simulink model "DCM_17_Series_18Ms_For_R_Discharge"  (R2019b)
settings: Solver=VariableStepAuto  StartTime=0.0  StopTime=30  RelTol=1e-3
model workspace (MAT data in the model file):
  Laf = 0.015
  Laf_2 = 0.00844
  Rarm = 0.0096
  angular_vel = 165
  angular_vel_1 = 175.405
  angular_vel_10 = 168.703
  angular_vel_11 = 168.598
  angular_vel_12 = 167.865
  angular_vel_13 = 167.132
  angular_vel_14 = 166.923
  angular_vel_15 = 165.666
  angular_vel_16 = 164.41
  angular_vel_2 = 173.625
  angular_vel_3 = 172.787
  angular_vel_4 = 170.902
  angular_vel_5 = 170.902
  angular_vel_6 = 169.96
  angular_vel_7 = 169.855
  angular_vel_8 = 169.122
libraries: powerlib x20, simulink x1
settings Model: OrderedModelArguments=off  Creator=Sy2  LastModifiedBy=Sy2
settings SolverCC: ZeroCrossAlgorithm=Adaptive
settings DebuggingCC: IgnoredZcDiagnostic=none

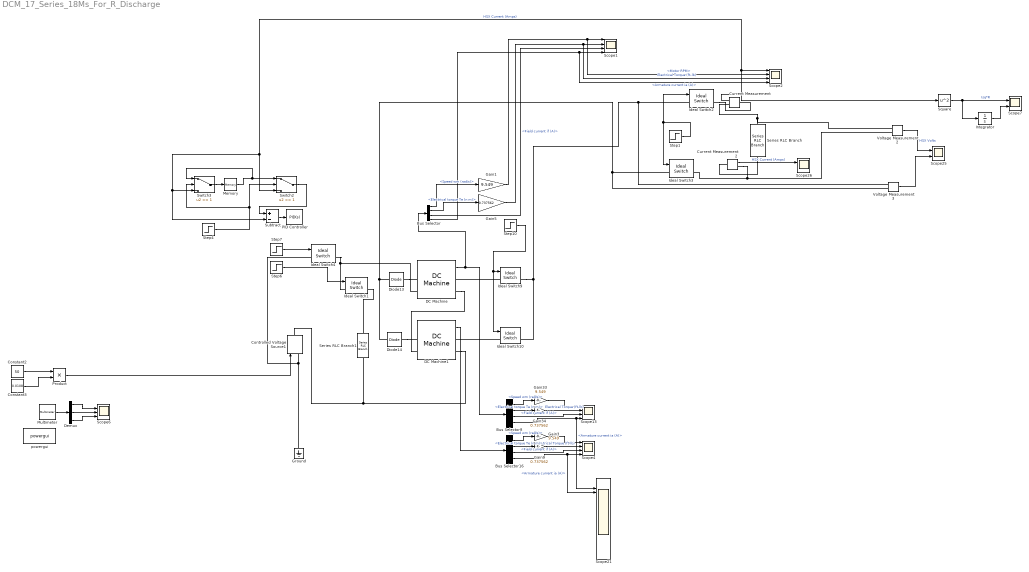
== system DCM_17_Series_18Ms_For_R_Discharge ==
  Bus Selector : BusSelector  OutputSignals=Speed wm (rad/s),Electrical torque Te (n m),Field current if (A),Armature current ia (A)
  Bus Selector16 : BusSelector  OutputSignals=Speed wm (rad/s),Electrical torque Te (n m),Field current if (A),Armature current ia (A)
  Bus Selector8 : BusSelector  OutputSignals=Speed wm (rad/s),Electrical torque Te (n m),Field current if (A),Armature current ia (A)
  Constant2 : Constant  Value=50
  Constant3 : Constant  Value=0.0108
  Controlled Voltage Source1 : powerlib/Electrical Sources/Controlled Voltage Source  Initialize=on  Source_Type=DC  Amplitude=0  Phase=0  Frequency=0  Measurements=Voltage
      settings: SourceProductName=Simscape Electrical
  Current Measurement : powerlib/Measurements/Current Measurement  PhasorSimulation=off  OutputType=Complex  PSBequivalent=0
      settings: SourceProductName=Simscape Electrical
  Current Measurement2 : powerlib/Measurements/Current Measurement  PhasorSimulation=off  OutputType=Complex  PSBequivalent=0
      settings: SourceProductName=Simscape Electrical
  DC Machine : powerlib/Machines/DC Machine  PresetModel=No  MechanicalLoad=Torque TL  FieldType=Wound  ShowDetailedParameters=on  MeasurementBus=off  RLa="[Rarm  0.002]"  RLf=[0.0054 0.0125]  Laf=Laf  MachineConstant=Torque constant (N.m/A)  Ke=1.8  Kt=1.8  J=137  Bm=0  Tf=0  w0=angular_vel  Ifinit=0  TsPowergui=0  TsBlock=-1
      settings: SourceProductName=Simscape Electrical
  DC Machine1 : powerlib/Machines/DC Machine  PresetModel=No  MechanicalLoad=Torque TL  FieldType=Wound  ShowDetailedParameters=on  MeasurementBus=off  RLa="[Rarm  0.002]"  RLf=[0.0054 0.0125]  Laf=Laf  MachineConstant=Torque constant (N.m/A)  Ke=1.8  Kt=1.8  J=137  Bm=0  Tf=0  w0=angular_vel  Ifinit=0  TsPowergui=0  TsBlock=-1
      settings: SourceProductName=Simscape Electrical
  Demux : Demux  Outputs=3
  Diode13 : powerlib/Power Electronics/Diode  Ron=0.0000001  Lon=0  Vf=0.8  IC=0  UseSnubber=0  Rs=500000  Cs=250e-9  Measurements=off
      settings: SourceProductName=Simscape Electrical
  Diode14 : powerlib/Power Electronics/Diode  Ron=0.001  Lon=0  Vf=0.8  IC=0  UseSnubber=0  Rs=500000  Cs=250e-9  Measurements=off
      settings: SourceProductName=Simscape Electrical
  Gain1 : Gain  Gain=9.549
  Gain3 : Gain  Gain=9.549
  Gain33 : Gain  Gain=9.549
  Gain34 : Gain  Gain=0.737562
  Gain5 : Gain  Gain=0.737562
  Gain9 : Gain  Gain=0.737562
  Ground : powerlib/Elements/Ground  LConnTagsString=a
      settings: SourceProductName=Simscape Electrical
  Ideal Switch{1..3,9..10} (5 alike) : powerlib/Power Electronics/Ideal Switch  Ron=0  Lon=0  IC=0  Rs=inf  Cs=0  Measurements=on
      settings: SourceProductName=Simscape Electrical
  Ideal Switch4 : powerlib/Power Electronics/Ideal Switch  Ron=0  Lon=0  IC=1  Rs=inf  Cs=0  Measurements=on
      settings: SourceProductName=Simscape Electrical
  Integrator : Integrator  ZeroCross=off
  Memory : Memory
  Multimeter : powerlib/Measurements/Multimeter  PhasorSimulation=off  OutputType=Complex  sel=[2 3 1]  L=3  Gain=[1 1 1]  yselected={'Usrc: Controlled Voltage Source1','Ib: Series RLC Branch1','Ub: Series RLC Branch1'};  PSBOutputType=1  PSBequivalent=0  AxesSetting=[0,0.1,-100,100]  Display=0  SavedBlockNames=-11
      settings: SourceProductName=Simscape Electrical
  PID Controller : simulink/Continuous/PID Controller  Controller=PID  Form=Parallel  TimeDomain=Continuous-time  SampleTime=-1  IntegratorMethod=Forward Euler  FilterMethod=Forward Euler  ControllerParametersSource=internal  P=10  I=7  D=1  UseFilter=on  N=100  TunerSelectOption=Transfer Function Based (PID Tuner App)  InitialConditionSource=internal  InitialConditionForIntegrator=0  InitialConditionForFilter=0  DifferentiatorICPrevScaledInput=0  ExternalReset=none  TrackingMode=off  Kt=1  LimitOutput=off  UpperSaturationLimit=inf  LowerSaturationLimit=-inf  LinearizeAsGain=on  AntiWindupMode=none  Kb=1  POutMin=[]  POutMax=[]  IOutMin=[]  IOutMax=[]  DOutMin=[]  DOutMax=[]  NOutMin=[]  NOutMax=[]  SumOutMin=[]  SumOutMax=[]  SaturationOutMin=[]  SaturationOutMax=[]  PParamMin=[]  PParamMax=[]  IParamMin=[]  IParamMax=[]  DParamMin=[]  DParamMax=[]  NParamMin=[]  NParamMax=[]  KbParamMin=[]  KbParamMax=[]  KtParamMin=[]  KtParamMax=[]  KbOutMin=[]  KbOutMax=[]  KtOutMin=[]  KtOutMax=[]  IntegratorOutMin=[]  IntegratorOutMax=[]  FilterOutMin=[]  FilterOutMax=[]  SumI1OutMin=[]  SumI1OutMax=[]  SumI2OutMin=[]  SumI2OutMax=[]  SumI3OutMin=[]  SumI3OutMax=[]  SumI4OutMin=[]  SumI4OutMax=[]  SumDOutMin=[]  SumDOutMax=[]  DifferentiatorOutMin=[]  DifferentiatorOutMax=[]  FilterDiffOutCoefMin=[]  FilterDiffOutCoefMax=[]  ReciprocalOutMin=[]  ReciprocalOutMax=[]  SumDenOutMin=[]  SumDenOutMax=[]  SumNumOutMin=[]  SumNumOutMax=[]  DivideOutMin=[]  DivideOutMax=[]  IntegratorContinuousStateAttributes=''  IntegratorStateMustResolveToSignalObject=off  IntegratorRTWStateStorageClass=Auto  FilterContinuousStateAttributes=''  FilterStateMustResolveToSignalObject=off  FilterRTWStateStorageClass=Auto  ParallelPVariant=InternalParameters  IdealPVariant=Disabled  IVariant=InternalParameters  DVariant=InternalParameters  IntegratorVariant=Continuous  SatVariant=Disabled  AWVariant=Passthrough  PCopyVariant=Disabled  TRVariant=Disabled  FdbkBlocksVariant=Forward  IdealPFdbkVariant=Disabled  SatFdbkVariant=Disabled  DerivativeFilterVariant=ContFilter  NVariant=InternalParameters  NCopyVariant=Disabled  FilterICVariant=InternalICsFilter  IntegratorICVariant=InternalICs  ExternalResetVariant=Disabled  TRSumVariant=Passthrough  SumFdbkVariant=Disabled  SumVariant=Sum_PID
  Product : Product
  Scope{1..2,4,13} (4 alike) : Scope  NumInputPorts=4
  Scope21 : Scope  NumInputPorts=16
  Scope25 : Scope  NumInputPorts=2
  Scope26 : Scope  NumInputPorts=2
  Scope6 : Scope  NumInputPorts=3
  Scope7 : Scope  NumInputPorts=2
  Series RLC Branch : powerlib/Elements/Series RLC Branch  LConnTagsString=__new0  RConnTagsString=__new0  BranchType=R  Resistance=0.1  Inductance=0.02  SetiL0=off  InitialCurrent=0  Capacitance=1e-6  Setx0=off  InitialVoltage=0  Measurements=None
      settings: SourceProductName=Simscape Electrical
  Series RLC Branch1 : powerlib/Elements/Series RLC Branch  Description=Field Dump Resistor  LConnTagsString=__new0  RConnTagsString=__new0  BranchType=R  Resistance=5  Inductance=1e-3  SetiL0=off  InitialCurrent=0  Capacitance=1e-6  Setx0=off  InitialVoltage=0  Measurements=Branch voltage and current
      settings: AttributesFormatString=%<Description>  SourceProductName=Simscape Electrical
  Square : Math  Operator=square  RndMeth=Zero  SaturateOnIntegerOverflow=on
  Step1 : Step  Time=12  SampleTime=0  VectorParams1D=off
  Step10 : Step  Time=12  SampleTime=0  VectorParams1D=off
  Step4 : Step  Time=12.72  SampleTime=0  VectorParams1D=off  ZeroCross=off
  Step6 : Step  Time=24  SampleTime=0  VectorParams1D=off  ZeroCross=off
  Step7 : Step  Time=24  Before=1  After=0  SampleTime=0  VectorParams1D=off  ZeroCross=off
  Subtract : Sum  Inputs=+-
  Switch2 : Switch  Threshold=1  ZeroCross=off
  Switch3 : Switch  Threshold=1  ZeroCross=off
  Voltage Measurement2 : powerlib/Measurements/Voltage Measurement  PhasorSimulation=off  OutputType=Complex  PSBequivalent=0
      settings: SourceProductName=Simscape Electrical
  Voltage Measurement3 : powerlib/Measurements/Voltage Measurement  PhasorSimulation=off  OutputType=Complex  PSBequivalent=0
      settings: SourceProductName=Simscape Electrical
  powergui : powerlib/powergui  Priority=1  SimulationMode=Continuous  SampleTime=50e-6  frequency=60  Iterations=50  frequencyindice=0  Pbase=100e6  ErrMax=1e-4  UnitsV=kV  UnitsW=MW  buscounter=0  FunctionMessages=off  echomessages=off  EnableUseOfTLC=off  CurrentSourceSwitches=off  DisableSnubberDevices=off  DisableRonSwitches=off  DisableVfSwitches=off  DisplayEquations=off  AutomaticDiscreteSolvers=off  SolverType=Tustin/Backward Euler (TBE)  Interpol=off  ExternalGateDelay=off  methode=off  Ts=100  x0status=blocks  SPID=on  SwTol=0  HookPort=off  NonlinearTolerance=1e-4  nMaxIteration=100  ContinueOnMaxIteration=off  RestoreLinks=warning  ResistiveCurrentMeasurement=off  Frange=[0:2:500]  Ylog=off  Xlog=on  ShowGrid=off  save=off  variable=ZData  structure=0  ZoomFFT=off  StartTime=0.0  cycles=1  DisplayStyle=1  fundamental=60  FreqAxis=off  MaxFrequency=1000  frequencyindicesteady=1  RmsSteady=1  display=off
      settings: SourceProductName=Simscape Electrical
  wires:
  Bus Selector/1 -> Gain1/1  "<Speed wm (rad/s)>"
  Bus Selector/3 -> Scope1/3  "<Field current if (A)>"
  Bus Selector/4 -> Scope2/4, Scope1/4  "<Armature current ia (A)>"
  Gain1/1 -> Scope1/1, Scope2/2  "<Motor RPM>"
  Step1/1 -> Ideal Switch2/1, Ideal Switch3/1
  Current Measurement/1 -> Square/1, Switch2/3, Switch3/3, Subtract/2, Scope2/1  "HSX Current (Amps)"
  Memory/1 -> Switch3/1, Switch2/1
  Subtract/1 -> PID Controller/1
  Constant2/1 -> Product/1
  Switch2/1 -> Subtract/1
  Step4/1 -> Switch2/2, Switch3/2
  Switch3/1 -> Memory/1
  Bus Selector/2 -> Gain5/1  "<Electrical torque Te (n m)>"
  Gain5/1 -> Scope2/3, Scope1/2  "Electrical Torque (ft-lb)"
  Square/1 -> Scope7/1, Integrator/1  "Isq*R"
  Integrator/1 -> Scope7/2
  Product/1 -> Controlled Voltage Source1/1
  Step6/1 -> Ideal Switch1/1
  Step7/1 -> Ideal Switch4/1
  Constant3/1 -> Product/2
  Demux/2 -> Scope6/2
  Multimeter/1 -> Demux/1
  Demux/1 -> Scope6/1
  Demux/3 -> Scope6/3
  Bus Selector8/3 -> Scope13/3  "<Field current if (A)>"
  Bus Selector8/2 -> Gain34/1  "<Electrical torque Te (n m)>"
  Gain34/1 -> Scope13/2  "Electrical Torque (ft-lb)"
  Bus Selector8/1 -> Gain33/1  "<Speed wm (rad/s)>"
  Gain33/1 -> Scope13/1
  Bus Selector8/4 -> Scope21/1, Scope13/4  "<Armature current ia (A)>"
  DC Machine/1 -> Bus Selector8/1, Bus Selector/1
  DC Machine1/1 -> Bus Selector16/1
  Gain3/1 -> Scope4/1
  Gain9/1 -> Scope4/2  "Electrical Torque (ft-lb)"
  Bus Selector16/1 -> Gain3/1  "<Speed wm (rad/s)>"
  Bus Selector16/3 -> Scope4/3  "<Field current if (A)>"
  Bus Selector16/2 -> Gain9/1  "<Electrical torque Te (n m)>"
  Bus Selector16/4 -> Scope21/2, Scope4/4  "<Armature current ia (A)>"
  Voltage Measurement2/1 -> Scope25/1  "HSX Volts"
  Current Measurement2/1 -> Scope26/1  "HSX Current (Amps)"
  Step10/1 -> Ideal Switch10/1, Ideal Switch9/1
  Voltage Measurement3/1 -> Scope25/2
  connections:
  Voltage Measurement2/LConn2 -- Ideal Switch3/RConn1 -- Current Measurement2/RConn1
  Ideal Switch9/RConn1 -- Ideal Switch10/RConn1 -- Ideal Switch2/LConn1 -- Voltage Measurement3/LConn1
  DC Machine/RConn2 -- DC Machine1/LConn2
  Controlled Voltage Source1/RConn1 -- DC Machine1/RConn2 -- Series RLC Branch1/RConn1
  DC Machine/LConn2 -- Ideal Switch4/RConn1 -- Ideal Switch1/LConn1
  Ideal Switch1/RConn1 -- Series RLC Branch1/LConn1
  Ideal Switch9/LConn1 -- DC Machine/RConn1
  Ideal Switch10/LConn1 -- DC Machine1/RConn1
  Diode14/RConn1 -- DC Machine1/LConn1
  Diode13/RConn1 -- DC Machine/LConn1
  Ground/LConn1 -- Controlled Voltage Source1/LConn1 -- Ideal Switch4/LConn1
  Ideal Switch2/RConn1 -- Current Measurement/LConn1
  Series RLC Branch/RConn1 -- Current Measurement2/LConn1
  Current Measurement/RConn1 -- Voltage Measurement2/LConn1 -- Series RLC Branch/LConn1
  Diode14/LConn1 -- Voltage Measurement3/LConn2 -- Ideal Switch3/LConn1 -- Diode13/LConn1
